simulink model "labTWOtaskTWO"  (R2023b)
settings: Solver=VariableStepAuto  StartTime=0.0  StopTime=10.0  RelTol=1e-3
libraries: dspfdesign x1
settings Model: Creator=omarf  LastModifiedBy=omarf

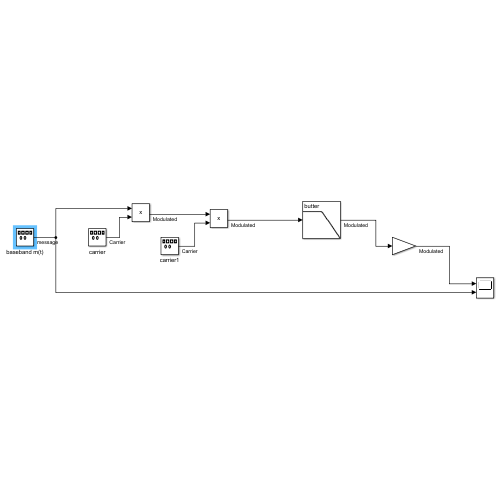
[thumbnail: Simulink's stored preview of the top-level diagram]
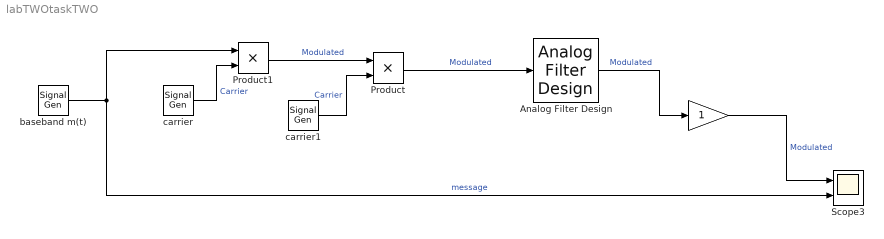
== system labTWOtaskTWO ==
  " " : Gain
  Analog Filter Design : dspfdesign/Analog Filter Design  method=Butterworth  filttype=Lowpass  N=8  Wlo=12600  Whi=80  Rp=2  Rs=40
  Product : Product
  Product1 : Product
  Scope3 : Scope  NumInputPorts=2
  baseband m(t) : SignalGenerator  Frequency=1000*2*pi  Units=rad/sec
  carrier : SignalGenerator  Frequency=20000*2*pi  Units=rad/sec
  carrier1 : SignalGenerator  Frequency=20000*2*pi  Units=rad/sec
  wires:
  Analog Filter Design/1 -> " "/1  "Modulated"
  Product/1 -> Analog Filter Design/1  "Modulated"
  baseband m(t)/1 -> Scope3/2, Product1/1  "message"
  carrier/1 -> Product1/2  "Carrier"
  Product1/1 -> Product/1  "Modulated"
  carrier1/1 -> Product/2  "Carrier"
  " "/1 -> Scope3/1  "Modulated"
